simulink library "libMdl_Imu"  (R2018a)
settings: Solver=VariableStepAuto  StartTime=0.0  StopTime=10.0  RelTol=1e-3
libraries: dspsrcs4 x1
settings Model: Creator=hwinter  LastModifiedBy=hwinter

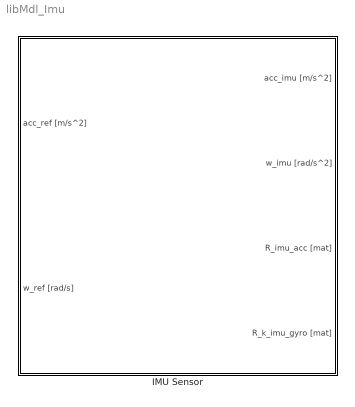
== system libMdl_Imu ==
  IMU Sensor : Subsystem  TreatAsAtomicUnit=on  SystemSampleTime=mv_T_imu  mask(IMU Sensor){mv_T_imu=-1, mv_sigma_imu_acc=[], mv_sigma_imu_gyro=[], mv_z_0_imu_acc=[], mv_z_0_imu_gyro=[], mv_seed_imu=[]}
      mask prompts: mv_T_imu "Sample time:"; mv_sigma_imu_acc "sigma_w_acc:"; mv_sigma_imu_gyro "sigma_w_gyro:"; mv_z_0_imu_acc "z_0_acc:"; mv_z_0_imu_gyro "z_0_gyro:"; mv_seed_imu "Seed:"
      mask help:
      | Sample Time:
      | Sample time of the block in seconds
      |
      | sigma_w_acc:
      | Standard deviation of the acceleration outputs
      | (format: [sigma_acc_x, sigma_acc_y, sigma_acc_z])
      |
      | sigma_w_gyro:
      | Standard deviation of the gyroscope outputs
      | (format: [sigma_gyro_roll, sigma_gyro_pitch, sigma_gyro_yaw])
      |
      | z_0_acc:
      | Initial accelerations
      | (format: [a_0_x, a_0_y, a_0_z])
      |
      | z_0_gyro:
      | Initial turn rates
      | (format: [w_0_roll, w_0_pitch, w_0_yaw]
      |
      | Seed:
      | Choose a seed for the random number generator
      mask init:
      | % parameter_field_name = 'RepMode';
      | % type_options = {'Repeatable','Not repeatable'};
      | % 
      | % block_handle = find_system(gcbh,'LookUnderMasks','all','Name','rnd_src');
      | % set_param(block_handle,parameter_field_name,type_options{mv_rep_mode});
      mask Display:
      | str1 = sprintf('\\color{black}{\\bf IMU}\n\n');
      | str2 = sprintf('Sample Time: %0.2f\n\n',mv_T_imu);
      | if length(mv_sigma_imu_acc) > 1
      |     str3 = sprintf('\\sigma_{x}: %0.2f\n',mv_sigma_imu_acc(1));
      |     str4 = sprintf('\\sigma_{y}: %0.2f\n',mv_sigma_imu_acc(2));
      |     str5 = sprintf('\\sigma_{z}: %0.2f\n',mv_sigma_imu_acc(3));
      | else
      |     str3 = sprintf('\\sigma_{x}: []\n');
      |     str4 = sprintf('\\sigma_{y}: []\n');
      |     str5 = sprintf('\\sigma_{z}: []\n');
      | end % if
      | if length(mv_sigma_imu_gyro) > 1
      |     str6 = sprintf('\\sigma_{roll}: %0.2f\n',mv_sigma_imu_gyro(1));
      |     str7 = sprintf('\\sigma_{pitch}: %0.2f\n',mv_sigma_imu_gyro(2));
      |     str8 = sprintf('\\sigma_{yaw}: %0.2f\n\n',mv_sigma_imu_gyro(3));
      | else
      |     str6 = sprintf('\\sigma_{roll}: []\n');
      |     str7 = sprintf('\\sigma_{pitch}: []\n');
      |     str8 = sprintf('\\sigma_{yaw}: []\n\n');
      | end % if
      | if length(mv_z_0_imu_acc) <= 3
      |     str9 = sprintf('z_0 (acc): %s\n',mat2str(mv_z_0_imu_acc,5));
      | else
      |     str9 = sprintf('z_0 (acc): [...]\n');
      | end % if
      | if length(mv_z_0_imu_gyro) <= 3
      |     str10 = sprintf('z_0 (gyro): %s\n\n',mat2str(mv_z_0_imu_gyro,5));
      | else
      |     str10 = sprintf('z_0 (gyro): [...]\n\n');
      | end % if
      | str11 = sprintf('Seed: %i\n\n',mv_seed_imu);
      | 
      | str = [str1,str2,str3,str4,str5,str6,str7,str8,str9,str10,str11];
      | 
      | text( 0.5,0.5, ...
      |       str, ...
      |       'horizontalAlignment', 'center', ...
      |       'texmode','on' ...
      |     )

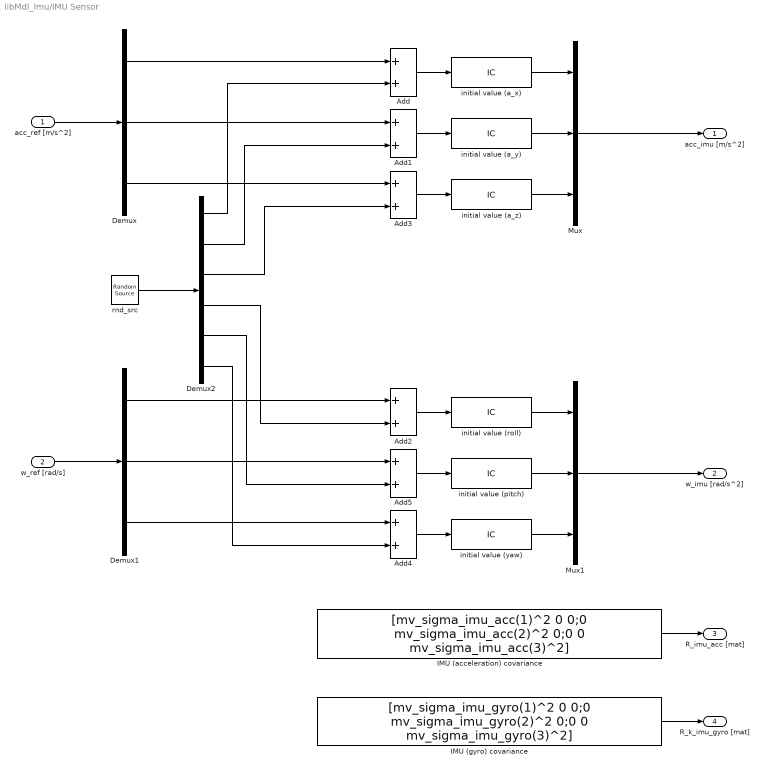
== system libMdl_Imu/IMU Sensor ==
  acc_ref [m/s^2] : Inport
  w_ref [rad/s] : Inport  Port=2
  Add{,1..5} (6 alike) : Sum
  Demux : Demux  Outputs=3
  Demux1 : Demux  Outputs=3
  Demux2 : Demux  Outputs=6
  IMU (acceleration) covariance : Constant  Value=[mv_sigma_imu_acc(1)^2 0 0;0 mv_sigma_imu_acc(2)^2 0;0 0 mv_sigma_imu_acc(3)^2]
  IMU (gyro) covariance : Constant  Value=[mv_sigma_imu_gyro(1)^2 0 0;0 mv_sigma_imu_gyro(2)^2 0;0 0 mv_sigma_imu_gyro(3)^2]
  Mux : Mux  Inputs=3
  Mux1 : Mux  Inputs=3
  initial value (a_x) : InitialCondition  Value=mv_z_0_imu_acc(1)
  initial value (a_y) : InitialCondition  Value=mv_z_0_imu_acc(2)
  initial value (a_z) : InitialCondition  Value=mv_z_0_imu_acc(3)
  initial value (pitch) : InitialCondition  Value=mv_z_0_imu_gyro(2)
  initial value (roll) : InitialCondition  Value=mv_z_0_imu_gyro(1)
  initial value (yaw) : InitialCondition  Value=mv_z_0_imu_gyro(3)
  rnd_src : dspsrcs4/Random Source  SrcType=Gaussian  NormMethod=Ziggurat  CltLength=12  MinVal=0  MaxVal=1  MeanVal=[0 0 0, 0 0 0]  VarVal=[mv_sigma_imu_acc.^2, mv_sigma_imu_gyro.^2]  RepMode=Specify seed  rawSeed=mv_seed_imu  IsInherit=on  SampMode=Discrete  SampTime=1  SampFrame=1  DataType=Double  OutComplex=Real  OutputFrames=off
  acc_imu [m/s^2] : Outport
  w_imu [rad/s^2] : Outport  Port=2
  R_imu_acc [mat] : Outport  Port=3
  R_k_imu_gyro [mat] : Outport  Port=4
  wires:
  Demux2/6 -> Add4/2
  Demux2/5 -> Add5/2
  Demux2/4 -> Add2/2
  Demux2/3 -> Add3/2
  Demux2/2 -> Add1/2
  Demux2/1 -> Add/2
  rnd_src/1 -> Demux2/1
  Mux/1 -> acc_imu [m/s^2]/1
  Demux/3 -> Add3/1
  Demux/2 -> Add1/1
  Demux/1 -> Add/1
  acc_ref [m/s^2]/1 -> Demux/1
  Add3/1 -> initial value (a_z)/1
  Add1/1 -> initial value (a_y)/1
  Add/1 -> initial value (a_x)/1
  IMU (gyro) covariance/1 -> R_k_imu_gyro [mat]/1
  Add4/1 -> initial value (yaw)/1
  Demux1/2 -> Add5/1
  Demux1/3 -> Add4/1
  Add2/1 -> initial value (roll)/1
  initial value (roll)/1 -> Mux1/1
  w_ref [rad/s]/1 -> Demux1/1
  initial value (yaw)/1 -> Mux1/3
  Add5/1 -> initial value (pitch)/1
  Mux1/1 -> w_imu [rad/s^2]/1
  initial value (pitch)/1 -> Mux1/2
  Demux1/1 -> Add2/1
  initial value (a_z)/1 -> Mux/3
  IMU (acceleration) covariance/1 -> R_imu_acc [mat]/1
  initial value (a_x)/1 -> Mux/1
  initial value (a_y)/1 -> Mux/2
